simulink model "Q5_L1"  (Simulink 9.2)
settings: Solver=VariableStepAuto  StartTime=0.0  StopTime=100  RelTol=1e-3
values from neighbouring files (symbols this model uses):
  b1 = input('Entre com o valor do atrito b1')    [Exercicio1.m]
  b2 = input('Entre com o valor do atrito b2')    [Exercicio1.m]
  k1 = input('Entre com o valor do k1')    [Exercicio1.m]
  k2 = input('Entre com o valor do k2')    [Exercicio1.m]
  m1 = sin(2*pi*fm1*t)    [FDM_senoides.m]
  m2 = input('Entre com o valor do massa m2')    [Exercicio1.m]    (also in FDM_senoides.m = sin(2*pi*fm2*t))
undefined symbols (not defined in the file or in its folder): F
settings Model: Creator=root  LastModifiedBy=root
settings DataIOCC: LimitDataPoints=off  SaveFormat=Dataset  SignalLoggingSaveFormat=Dataset
settings OptimizationCC: LifeSpan=auto
settings DebuggingCC: UnderspecifiedInitializationDetection=Simplified  MergeDetectMultiDrivingBlocksExec=error  FcnCallInpInsideContextMsg=error  StateNameClashWarn=none  SFUnexpectedBacktrackingDiag=error  SFNoUnconditionalDefaultTransitionDiag=error  SFExecutionAtInitializationDiag=warning
settings HardwareCC: ProdBitPerPointer=64  ProdBitPerSizeT=64  ProdBitPerPtrDiffT=64  ProdLargestAtomicFloat=Float  ProdIntDivRoundTo=Zero  ProdEndianess=LittleEndian  ProdWordSize=64  ProdHWDeviceType=Intel->x86-64 (Windows64)
settings ModelReferenceCC: PropagateSignalLabelsOutOfModel=on
settings SFSimCC: SimUseLocalCustomCode=on
settings RTWCC: RTWUseLocalCustomCode=on
settings CodeAppCC: StateflowObjectComments=off
settings GRTTargetCC: TargetLangStandard=C99 (ISO)  GeneratePreprocessorConditionals=Use local settings  CombineOutputUpdateFcns=on  GRTInterface=off
settings ConfigComp: CovMetricSettings=dwe  CovHtmlReporting=off  CovSaveCumulativeToWorkspaceVar=off  CovSaveSingleToWorkspaceVar=off  CovExternalEMLEnable=on

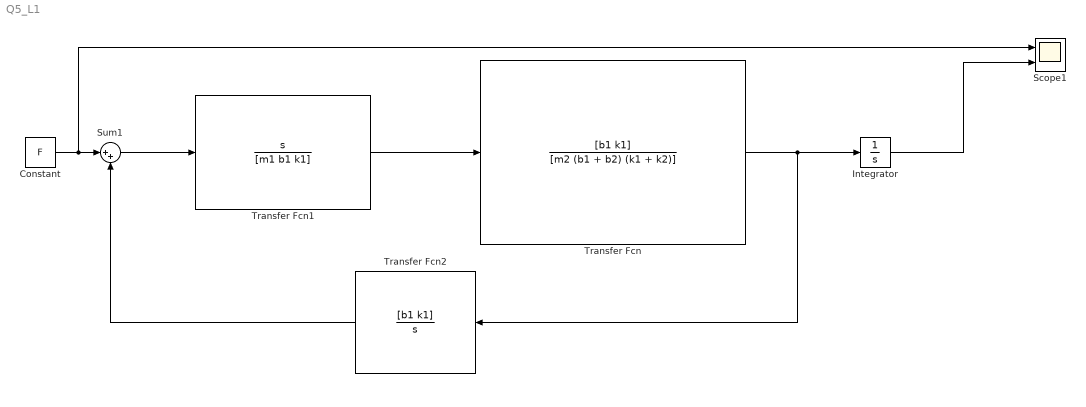
== system Q5_L1 ==
  Constant : Constant  Value=F
  Integrator : Integrator
  Scope1 : Scope  NumInputPorts=2
  Sum1 : Sum  Inputs=|++
  Transfer Fcn : TransferFcn  Numerator=[b1 k1]  Denominator=[m2 (b1 + b2) (k1 + k2)]
  Transfer Fcn1 : TransferFcn  Numerator=[1 0]  Denominator=[m1 b1 k1]
  Transfer Fcn2 : TransferFcn  Numerator=[b1 k1]  Denominator=[1 0]
  wires:
  Transfer Fcn1/1 -> Transfer Fcn/1
  Transfer Fcn/1 -> Transfer Fcn2/1, Integrator/1
  Sum1/1 -> Transfer Fcn1/1
  Constant/1 -> Scope1/1, Sum1/1
  Transfer Fcn2/1 -> Sum1/2
  Integrator/1 -> Scope1/2
